simulink library "halout"  (R2021b)
settings: Solver=VariableStepAuto  StartTime=0.0  StopTime=10.0  RelTol=1e-3
undefined symbols (not defined in the file): C_TASK_5MS_S, FALSE, KHAL_CAN1TxReq_flg, KHAL_CAN2TxReq_flg, KHAL_CAN3FD3VCU1toNIDECTxReq_flg, KHAL_CAN3FD3VCU1TxReq_flg, KHAL_CAN3FD3VCU2E2E_flg, KHAL_CAN3FD3VCU2toNIDECE2E_flg, KHAL_CAN3FD3VCU2toNIDECTxReq_flg, KHAL_CAN3FD3VCU2TxReq_flg, KHAL_CAN3TxReq_flg, KHAL_CAN4FD4CE1000E2E_flg, KHAL_CAN4FD4CE1000TxReq_flg, KHAL_CAN4TxReq_flg, KHAL_CAN5TxReq_flg, KHAL_CAN7TxReq_flg, ONE_INT, TRUE, ZERO_INT
libraries: FVT_lib x258, simulink x115
(part 9 of 17)

== system halout/HAL_OUT/CAN5/FD5_CE100_0_0x118 ==
  BSCP_outputs : Inport  OutDataTypeStr=Bus: BSCP_outputs
  BOUTP_outputs : Inport  Port=2  OutDataTypeStr=Bus: BOUTP_outputs
  AllDoorSW : Subsystem
  AntitheftSta : Subsystem
  BCMDoorLockSta : Subsystem
  CCUACLampSts : Subsystem
  CCUCbnPreACWkSts : Subsystem
  CCUCbnPreEstimdTi : Subsystem
  CCUCbnPreSts : Subsystem
  FDTBOXDTCDataErr : Subsystem
  FDTBOXDTCDataSta : Subsystem
  FDTBOXVehDataErr : Subsystem
  FDTBOXVehDataSta : Subsystem
  Ground{,1..13} (14 alike) : Ground
  HoodSW : Subsystem
  LowSOCWarn : Subsystem
  PwrSta : Subsystem
  ReVehThdChkSta : Subsystem
  ShiftGearPosn : Subsystem
  TCountSta : Subsystem
  TailgateRemote : Subsystem
  TailgateSW : Subsystem
  VehMalfunLevel : Subsystem
  bus_creator : BusCreator  Inputs=20  OutDataTypeStr=Bus: DT_CAN5_SG_FD5_CE100_0  NonVirtualBus=on
  bus_selector : BusSelector  OutputSignals=VOUTP_CCUACLampSts_flg
  bus_selector1 : BusSelector  OutputSignals=VOUTP_LowSOCWarn_enum
  bus_selector2 : BusSelector  OutputSignals=VOUTP_PowerSta_enum
  bus_selector3 : BusSelector  OutputSignals=VOUTP_ReVehThdChkSta_enum
  bus_selector4 : BusSelector  OutputSignals=VOUTP_ShiftGearPosn_enum
  bus_selector5 : BusSelector  OutputSignals=VOUTP_TCountSta_enum
  FD5_CE100_0 : Outport
  wires:
  BSCP_outputs/1 -> [BSCP_outputs]
  BOUTP_outputs/1 -> [BOUTP_outputs]
  [CAN5_AllDoorSW] -> bus_creator/1  "CAN5_AllDoorSW"
  [CAN5_AntitheftSta] -> bus_creator/2  "CAN5_AntitheftSta"
  [CAN5_BCM_DoorLock_Sta] -> bus_creator/3  "CAN5_BCM_DoorLock_Sta"
  [CAN5_CCU_ACLampSts] -> bus_creator/4  "CAN5_CCU_ACLampSts"
  [CAN5_CCU_CbnPreACWkSts] -> bus_creator/5  "CAN5_CCU_CbnPreACWkSts"
  [CAN5_CCU_CbnPreEstimdTi] -> bus_creator/6  "CAN5_CCU_CbnPreEstimdTi"
  [CAN5_CCU_CbnPreSts] -> bus_creator/7  "CAN5_CCU_CbnPreSts"
  [CAN5_FD_TBOX_DTCData_Err] -> bus_creator/8  "CAN5_FD_TBOX_DTCData_Err"
  [CAN5_FD_TBOX_DTCData_Sta] -> bus_creator/9  "CAN5_FD_TBOX_DTCData_Sta"
  [CAN5_FD_TBOX_VehData_Err] -> bus_creator/10  "CAN5_FD_TBOX_VehData_Err"
  [CAN5_FD_TBOX_VehData_Sta] -> bus_creator/11  "CAN5_FD_TBOX_VehData_Sta"
  [CAN5_HoodSW] -> bus_creator/12  "CAN5_HoodSW"
  [CAN5_LowSOCWarn] -> bus_creator/13  "CAN5_LowSOCWarn"
  [CAN5_PwrSta] -> bus_creator/14  "CAN5_PwrSta"
  [CAN5_Re_VehThdChkSta] -> bus_creator/15  "CAN5_Re_VehThdChkSta"
  [CAN5_ShiftGearPosn] -> bus_creator/16  "CAN5_ShiftGearPosn"
  [CAN5_TCountSta] -> bus_creator/17  "CAN5_TCountSta"
  [CAN5_TailgateRemote] -> bus_creator/18  "CAN5_TailgateRemote"
  [CAN5_Tailgate_SW] -> bus_creator/19  "CAN5_Tailgate_SW"
  [CAN5_VehMalfunLevel] -> bus_creator/20  "CAN5_VehMalfunLevel"
  bus_creator/1 -> FD5_CE100_0/1
  AllDoorSW/1(CAN5_AllDoorSW) -> [CAN5_AllDoorSW]
  AntitheftSta/1(CAN5_AntitheftSta) -> [CAN5_AntitheftSta]
  BCMDoorLockSta/1(CAN5_BCM_DoorLock_Sta) -> [CAN5_BCM_DoorLock_Sta]
  CCUACLampSts/1(CAN5_CCU_ACLampSts) -> [CAN5_CCU_ACLampSts]
  CCUCbnPreACWkSts/1(CAN5_CCU_CbnPreACWkSts) -> [CAN5_CCU_CbnPreACWkSts]
  CCUCbnPreEstimdTi/1(CAN5_CCU_CbnPreEstimdTi) -> [CAN5_CCU_CbnPreEstimdTi]
  CCUCbnPreSts/1(CAN5_CCU_CbnPreSts) -> [CAN5_CCU_CbnPreSts]
  FDTBOXDTCDataErr/1(CAN5_FD_TBOX_DTCData_Err) -> [CAN5_FD_TBOX_DTCData_Err]
  FDTBOXDTCDataSta/1(CAN5_FD_TBOX_DTCData_Sta) -> [CAN5_FD_TBOX_DTCData_Sta]
  FDTBOXVehDataErr/1(CAN5_FD_TBOX_VehData_Err) -> [CAN5_FD_TBOX_VehData_Err]
  FDTBOXVehDataSta/1(CAN5_FD_TBOX_VehData_Sta) -> [CAN5_FD_TBOX_VehData_Sta]
  HoodSW/1(CAN5_HoodSW) -> [CAN5_HoodSW]
  LowSOCWarn/1(CAN5_LowSOCWarn) -> [CAN5_LowSOCWarn]
  PwrSta/1(CAN5_PwrSta) -> [CAN5_PwrSta]
  ReVehThdChkSta/1(CAN5_Re_VehThdChkSta) -> [CAN5_Re_VehThdChkSta]
  ShiftGearPosn/1(CAN5_ShiftGearPosn) -> [CAN5_ShiftGearPosn]
  TCountSta/1(CAN5_TCountSta) -> [CAN5_TCountSta]
  TailgateRemote/1(CAN5_TailgateRemote) -> [CAN5_TailgateRemote]
  TailgateSW/1(CAN5_Tailgate_SW) -> [CAN5_Tailgate_SW]
  VehMalfunLevel/1(CAN5_VehMalfunLevel) -> [CAN5_VehMalfunLevel]
  Ground/1 -> AllDoorSW/1(AllDoorSW)
  Ground1/1 -> AntitheftSta/1(AntitheftSta)
  Ground2/1 -> BCMDoorLockSta/1(BCMDoorLockSta)
  bus_selector/1 -> CCUACLampSts/1(CCUACLampSts)  "<VOUTP_CCUACLampSts_flg>"
  [BOUTP_outputs] -> bus_selector/1
  Ground3/1 -> CCUCbnPreACWkSts/1(CCUCbnPreACWkSts)
  Ground4/1 -> CCUCbnPreEstimdTi/1(CCUCbnPreEstimdTi)
  Ground5/1 -> CCUCbnPreSts/1(CCUCbnPreSts)
  Ground6/1 -> FDTBOXDTCDataErr/1(FDTBOXDTCDataErr)
  Ground7/1 -> FDTBOXDTCDataSta/1(FDTBOXDTCDataSta)
  Ground8/1 -> FDTBOXVehDataErr/1(FDTBOXVehDataErr)
  Ground9/1 -> FDTBOXVehDataSta/1(FDTBOXVehDataSta)
  Ground10/1 -> HoodSW/1(HoodSW)
  bus_selector1/1 -> LowSOCWarn/1(LowSOCWarn)  "<VOUTP_LowSOCWarn_enum>"
  [BOUTP_outputs] -> bus_selector1/1
  bus_selector2/1 -> PwrSta/1(PwrSta)  "<VOUTP_PowerSta_enum>"
  [BOUTP_outputs] -> bus_selector2/1
  bus_selector3/1 -> ReVehThdChkSta/1(ReVehThdChkSta)  "<VOUTP_ReVehThdChkSta_enum>"
  [BOUTP_outputs] -> bus_selector3/1
  bus_selector4/1 -> ShiftGearPosn/1(ShiftGearPosn)  "<VOUTP_ShiftGearPosn_enum>"
  [BOUTP_outputs] -> bus_selector4/1
  bus_selector5/1 -> TCountSta/1(TCountSta)  "<VOUTP_TCountSta_enum>"
  [BOUTP_outputs] -> bus_selector5/1
  Ground11/1 -> TailgateRemote/1(TailgateRemote)
  Ground12/1 -> TailgateSW/1(TailgateSW)
  Ground13/1 -> VehMalfunLevel/1(VehMalfunLevel)

== system halout/HAL_OUT/CAN5/FD5_Debug1_0x4D0 ==
  BSCP_outputs : Inport  OutDataTypeStr=Bus: BSCP_outputs
  BOUTP_outputs : Inport  Port=2  OutDataTypeStr=Bus: BOUTP_outputs
  ID1ALTU : Subsystem
  ID1LocALTU : Subsystem
  ID1messageALTU : Subsystem
  ID2ALTU : Subsystem
  ID2LocALTU : Subsystem
  ID2messageALTU : Subsystem
  ID3ALTU : Subsystem
  ID3LocALTU : Subsystem
  ID3messageALTU : Subsystem
  ID4ALTU : Subsystem
  ID4LocALTU : Subsystem
  ID4messageALTU : Subsystem
  IDinALTU : Subsystem
  LFSensorMode : Subsystem
  LRSensorMode : Subsystem
  RFFATALTU : Subsystem
  RFSensorMode : Subsystem
  RRSensorMode : Subsystem
  S1WheelDebugALTU : Subsystem
  S2WheelDebugALTU : Subsystem
  S3WheelDebugALTU : Subsystem
  S4WheelDebugALTU : Subsystem
  bus_creator : BusCreator  Inputs=22  OutDataTypeStr=Bus: DT_CAN5_SG_FD5_Debug1  NonVirtualBus=on
  bus_selector : BusSelector  OutputSignals=VOUTP_S1ID_raw32
  bus_selector1 : BusSelector  OutputSignals=VOUTP_S1L_enum
  bus_selector10 : BusSelector  OutputSignals=VOUTP_S4L_enum
  bus_selector11 : BusSelector  OutputSignals=VOUTP_ID4messageALTU_raw8
  bus_selector12 : BusSelector  OutputSignals=VOUTP_IDin_raw32
  bus_selector13 : BusSelector  OutputSignals=VOUTP_LFSensorMode_flg
  bus_selector14 : BusSelector  OutputSignals=VOUTP_LRSensorMode_flg
  bus_selector15 : BusSelector  OutputSignals=VOUTP_RFSensorMode_flg
  bus_selector16 : BusSelector  OutputSignals=VOUTP_FAT_flg
  bus_selector17 : BusSelector  OutputSignals=VOUTP_RRSensorMode_flg
  bus_selector18 : BusSelector  OutputSignals=VOUTP_S1WheelDebugALTU_pct
  bus_selector19 : BusSelector  OutputSignals=VOUTP_S2WheelDebugALTU_pct
  bus_selector2 : BusSelector  OutputSignals=VOUTP_ID1messageALTU_raw8
  bus_selector20 : BusSelector  OutputSignals=VOUTP_S3WheelDebugALTU_pct
  bus_selector21 : BusSelector  OutputSignals=VOUTP_S4WheelDebugALTU_pct
  bus_selector3 : BusSelector  OutputSignals=VOUTP_S2ID_raw32
  bus_selector4 : BusSelector  OutputSignals=VOUTP_S2L_enum
  bus_selector5 : BusSelector  OutputSignals=VOUTP_ID2messageALTU_raw8
  bus_selector6 : BusSelector  OutputSignals=VOUTP_S3ID_raw32
  bus_selector7 : BusSelector  OutputSignals=VOUTP_S3L_enum
  bus_selector8 : BusSelector  OutputSignals=VOUTP_ID3messageALTU_raw8
  bus_selector9 : BusSelector  OutputSignals=VOUTP_S4ID_raw32
  FD5_Debug1 : Outport
  wires:
  BSCP_outputs/1 -> [BSCP_outputs]
  BOUTP_outputs/1 -> [BOUTP_outputs]
  [CAN5_ID1_ALTU] -> bus_creator/1  "CAN5_ID1_ALTU"
  [CAN5_ID1_Loc_ALTU] -> bus_creator/2  "CAN5_ID1_Loc_ALTU"
  [CAN5_ID1_message_ALTU] -> bus_creator/3  "CAN5_ID1_message_ALTU"
  [CAN5_ID2_ALTU] -> bus_creator/4  "CAN5_ID2_ALTU"
  [CAN5_ID2_Loc_ALTU] -> bus_creator/5  "CAN5_ID2_Loc_ALTU"
  [CAN5_ID2_message_ALTU] -> bus_creator/6  "CAN5_ID2_message_ALTU"
  [CAN5_ID3_ALTU] -> bus_creator/7  "CAN5_ID3_ALTU"
  [CAN5_ID3_Loc_ALTU] -> bus_creator/8  "CAN5_ID3_Loc_ALTU"
  [CAN5_ID3_message_ALTU] -> bus_creator/9  "CAN5_ID3_message_ALTU"
  [CAN5_ID4_ALTU] -> bus_creator/10  "CAN5_ID4_ALTU"
  [CAN5_ID4_Loc_ALTU] -> bus_creator/11  "CAN5_ID4_Loc_ALTU"
  [CAN5_ID4_message_ALTU] -> bus_creator/12  "CAN5_ID4_message_ALTU"
  [CAN5_IDin_ALTU] -> bus_creator/13  "CAN5_IDin_ALTU"
  [CAN5_LFSensorMode] -> bus_creator/14  "CAN5_LFSensorMode"
  [CAN5_LRSensorMode] -> bus_creator/15  "CAN5_LRSensorMode"
  [CAN5_RFSensorMode] -> bus_creator/16  "CAN5_RFSensorMode"
  [CAN5_RF_FAT_ALTU] -> bus_creator/17  "CAN5_RF_FAT_ALTU"
  [CAN5_RRSensorMode] -> bus_creator/18  "CAN5_RRSensorMode"
  [CAN5_S1WheelDebug_ALTU] -> bus_creator/19  "CAN5_S1WheelDebug_ALTU"
  [CAN5_S2WheelDebug_ALTU] -> bus_creator/20  "CAN5_S2WheelDebug_ALTU"
  [CAN5_S3WheelDebug_ALTU] -> bus_creator/21  "CAN5_S3WheelDebug_ALTU"
  [CAN5_S4WheelDebug_ALTU] -> bus_creator/22  "CAN5_S4WheelDebug_ALTU"
  bus_creator/1 -> FD5_Debug1/1
  ID1ALTU/1(CAN5_ID1_ALTU) -> [CAN5_ID1_ALTU]
  ID1LocALTU/1(CAN5_ID1_Loc_ALTU) -> [CAN5_ID1_Loc_ALTU]
  ID1messageALTU/1(CAN5_ID1_message_ALTU) -> [CAN5_ID1_message_ALTU]
  ID2ALTU/1(CAN5_ID2_ALTU) -> [CAN5_ID2_ALTU]
  ID2LocALTU/1(CAN5_ID2_Loc_ALTU) -> [CAN5_ID2_Loc_ALTU]
  ID2messageALTU/1(CAN5_ID2_message_ALTU) -> [CAN5_ID2_message_ALTU]
  ID3ALTU/1(CAN5_ID3_ALTU) -> [CAN5_ID3_ALTU]
  ID3LocALTU/1(CAN5_ID3_Loc_ALTU) -> [CAN5_ID3_Loc_ALTU]
  ID3messageALTU/1(CAN5_ID3_message_ALTU) -> [CAN5_ID3_message_ALTU]
  ID4ALTU/1(CAN5_ID4_ALTU) -> [CAN5_ID4_ALTU]
  ID4LocALTU/1(CAN5_ID4_Loc_ALTU) -> [CAN5_ID4_Loc_ALTU]
  ID4messageALTU/1(CAN5_ID4_message_ALTU) -> [CAN5_ID4_message_ALTU]
  IDinALTU/1(CAN5_IDin_ALTU) -> [CAN5_IDin_ALTU]
  LFSensorMode/1(CAN5_LFSensorMode) -> [CAN5_LFSensorMode]
  LRSensorMode/1(CAN5_LRSensorMode) -> [CAN5_LRSensorMode]
  RFSensorMode/1(CAN5_RFSensorMode) -> [CAN5_RFSensorMode]
  RFFATALTU/1(CAN5_RF_FAT_ALTU) -> [CAN5_RF_FAT_ALTU]
  RRSensorMode/1(CAN5_RRSensorMode) -> [CAN5_RRSensorMode]
  S1WheelDebugALTU/1(CAN5_S1WheelDebug_ALTU) -> [CAN5_S1WheelDebug_ALTU]
  S2WheelDebugALTU/1(CAN5_S2WheelDebug_ALTU) -> [CAN5_S2WheelDebug_ALTU]
  S3WheelDebugALTU/1(CAN5_S3WheelDebug_ALTU) -> [CAN5_S3WheelDebug_ALTU]
  S4WheelDebugALTU/1(CAN5_S4WheelDebug_ALTU) -> [CAN5_S4WheelDebug_ALTU]
  bus_selector/1 -> ID1ALTU/1(ID1ALTU)  "<VOUTP_S1ID_raw32>"
  [BOUTP_outputs] -> bus_selector/1
  bus_selector1/1 -> ID1LocALTU/1(ID1LocALTU)  "<VOUTP_S1L_enum>"
  [BOUTP_outputs] -> bus_selector1/1
  bus_selector2/1 -> ID1messageALTU/1(ID1messageALTU)  "<VOUTP_ID1messageALTU_raw8>"
  [BOUTP_outputs] -> bus_selector2/1
  bus_selector3/1 -> ID2ALTU/1(ID2ALTU)  "<VOUTP_S2ID_raw32>"
  [BOUTP_outputs] -> bus_selector3/1
  bus_selector4/1 -> ID2LocALTU/1(ID2LocALTU)  "<VOUTP_S2L_enum>"
  [BOUTP_outputs] -> bus_selector4/1
  bus_selector5/1 -> ID2messageALTU/1(ID2messageALTU)  "<VOUTP_ID2messageALTU_raw8>"
  [BOUTP_outputs] -> bus_selector5/1
  bus_selector6/1 -> ID3ALTU/1(ID3ALTU)  "<VOUTP_S3ID_raw32>"
  [BOUTP_outputs] -> bus_selector6/1
  bus_selector7/1 -> ID3LocALTU/1(ID3LocALTU)  "<VOUTP_S3L_enum>"
  [BOUTP_outputs] -> bus_selector7/1
  bus_selector8/1 -> ID3messageALTU/1(ID3messageALTU)  "<VOUTP_ID3messageALTU_raw8>"
  [BOUTP_outputs] -> bus_selector8/1
  bus_selector9/1 -> ID4ALTU/1(ID4ALTU)  "<VOUTP_S4ID_raw32>"
  [BOUTP_outputs] -> bus_selector9/1
  bus_selector10/1 -> ID4LocALTU/1(ID4LocALTU)  "<VOUTP_S4L_enum>"
  [BOUTP_outputs] -> bus_selector10/1
  bus_selector11/1 -> ID4messageALTU/1(ID4messageALTU)  "<VOUTP_ID4messageALTU_raw8>"
  [BOUTP_outputs] -> bus_selector11/1
  bus_selector12/1 -> IDinALTU/1(IDinALTU)  "<VOUTP_IDin_raw32>"
  [BOUTP_outputs] -> bus_selector12/1
  bus_selector13/1 -> LFSensorMode/1(LFSensorMode)  "<VOUTP_LFSensorMode_flg>"
  [BOUTP_outputs] -> bus_selector13/1
  bus_selector14/1 -> LRSensorMode/1(LRSensorMode)  "<VOUTP_LRSensorMode_flg>"
  [BOUTP_outputs] -> bus_selector14/1
  bus_selector15/1 -> RFSensorMode/1(RFSensorMode)  "<VOUTP_RFSensorMode_flg>"
  [BOUTP_outputs] -> bus_selector15/1
  bus_selector16/1 -> RFFATALTU/1(RFFATALTU)  "<VOUTP_FAT_flg>"
  [BOUTP_outputs] -> bus_selector16/1
  bus_selector17/1 -> RRSensorMode/1(RRSensorMode)  "<VOUTP_RRSensorMode_flg>"
  [BOUTP_outputs] -> bus_selector17/1
  bus_selector18/1 -> S1WheelDebugALTU/1(S1WheelDebugALTU)  "<VOUTP_S1WheelDebugALTU_pct>"
  [BOUTP_outputs] -> bus_selector18/1
  bus_selector19/1 -> S2WheelDebugALTU/1(S2WheelDebugALTU)  "<VOUTP_S2WheelDebugALTU_pct>"
  [BOUTP_outputs] -> bus_selector19/1
  bus_selector20/1 -> S3WheelDebugALTU/1(S3WheelDebugALTU)  "<VOUTP_S3WheelDebugALTU_pct>"
  [BOUTP_outputs] -> bus_selector20/1
  bus_selector21/1 -> S4WheelDebugALTU/1(S4WheelDebugALTU)  "<VOUTP_S4WheelDebugALTU_pct>"
  [BOUTP_outputs] -> bus_selector21/1

== system halout/HAL_OUT/CAN5/GW5_CE100_0_0x1C5 ==
  BSCP_outputs : Inport  OutDataTypeStr=Bus: BSCP_outputs
  BOUTP_outputs : Inport  Port=2  OutDataTypeStr=Bus: BOUTP_outputs
  BrkSwSta : Subsystem
  CrashOutputSts : Subsystem
  Ground{,1..10} (11 alike) : Ground
  PTGActiveSta : Subsystem
  PTGExist : Subsystem
  PTGSysSta : Subsystem
  VehSpeed : Subsystem
  ZLAPMWinLFOpenedSta : Subsystem
  ZLAPMWinLROpenedSta : Subsystem
  ZRAPMWinRFOpenedSta : Subsystem
  ZRAPMWinRROpenedSta : Subsystem
  ZRPTGActiveSta : Subsystem
  ZRPTGExistSta : Subsystem
  ZRPTGSysSta : Subsystem
  bus_creator : BusCreator  Inputs=13  OutDataTypeStr=Bus: DT_CAN5_SG_GW5_CE100_0  NonVirtualBus=on
  bus_selector : BusSelector  OutputSignals=VOUTP_SCPBrkSwSta_flg
  bus_selector1 : BusSelector  OutputSignals=VOUTP_Vehspeed_kph
  GW5_CE100_0 : Outport
  wires:
  BSCP_outputs/1 -> [BSCP_outputs]
  BOUTP_outputs/1 -> [BOUTP_outputs]
  [CAN5_BrkSw_Sta] -> bus_creator/1  "CAN5_BrkSw_Sta"
  [CAN5_CrashOutputSts] -> bus_creator/2  "CAN5_CrashOutputSts"
  [CAN5_PTG_Active_Sta] -> bus_creator/3  "CAN5_PTG_Active_Sta"
  [CAN5_PTG_Exist] -> bus_creator/4  "CAN5_PTG_Exist"
  [CAN5_PTG_Sys_Sta] -> bus_creator/5  "CAN5_PTG_Sys_Sta"
  [CAN5_VehSpeed] -> bus_creator/6  "CAN5_VehSpeed"
  [CAN5_ZL_APM_WinLFOpened_Sta] -> bus_creator/7  "CAN5_ZL_APM_WinLFOpened_Sta"
  [CAN5_ZL_APM_WinLROpened_Sta] -> bus_creator/8  "CAN5_ZL_APM_WinLROpened_Sta"
  [CAN5_ZR_APM_WinRFOpened_Sta] -> bus_creator/9  "CAN5_ZR_APM_WinRFOpened_Sta"
  [CAN5_ZR_APM_WinRROpened_Sta] -> bus_creator/10  "CAN5_ZR_APM_WinRROpened_Sta"
  [CAN5_ZR_PTG_Active_Sta] -> bus_creator/11  "CAN5_ZR_PTG_Active_Sta"
  [CAN5_ZR_PTG_Exist_Sta] -> bus_creator/12  "CAN5_ZR_PTG_Exist_Sta"
  [CAN5_ZR_PTG_Sys_Sta] -> bus_creator/13  "CAN5_ZR_PTG_Sys_Sta"
  bus_creator/1 -> GW5_CE100_0/1
  BrkSwSta/1(CAN5_BrkSw_Sta) -> [CAN5_BrkSw_Sta]
  CrashOutputSts/1(CAN5_CrashOutputSts) -> [CAN5_CrashOutputSts]
  PTGActiveSta/1(CAN5_PTG_Active_Sta) -> [CAN5_PTG_Active_Sta]
  PTGExist/1(CAN5_PTG_Exist) -> [CAN5_PTG_Exist]
  PTGSysSta/1(CAN5_PTG_Sys_Sta) -> [CAN5_PTG_Sys_Sta]
  VehSpeed/1(CAN5_VehSpeed) -> [CAN5_VehSpeed]
  ZLAPMWinLFOpenedSta/1(CAN5_ZL_APM_WinLFOpened_Sta) -> [CAN5_ZL_APM_WinLFOpened_Sta]
  ZLAPMWinLROpenedSta/1(CAN5_ZL_APM_WinLROpened_Sta) -> [CAN5_ZL_APM_WinLROpened_Sta]
  ZRAPMWinRFOpenedSta/1(CAN5_ZR_APM_WinRFOpened_Sta) -> [CAN5_ZR_APM_WinRFOpened_Sta]
  ZRAPMWinRROpenedSta/1(CAN5_ZR_APM_WinRROpened_Sta) -> [CAN5_ZR_APM_WinRROpened_Sta]
  ZRPTGActiveSta/1(CAN5_ZR_PTG_Active_Sta) -> [CAN5_ZR_PTG_Active_Sta]
  ZRPTGExistSta/1(CAN5_ZR_PTG_Exist_Sta) -> [CAN5_ZR_PTG_Exist_Sta]
  ZRPTGSysSta/1(CAN5_ZR_PTG_Sys_Sta) -> [CAN5_ZR_PTG_Sys_Sta]
  bus_selector/1 -> BrkSwSta/1(BrkSwSta)  "<VOUTP_SCPBrkSwSta_flg>"
  [BOUTP_outputs] -> bus_selector/1
  Ground/1 -> CrashOutputSts/1(CrashOutputSts)
  Ground1/1 -> PTGActiveSta/1(PTGActiveSta)
  Ground2/1 -> PTGExist/1(PTGExist)
  Ground3/1 -> PTGSysSta/1(PTGSysSta)
  bus_selector1/1 -> VehSpeed/1(VehSpeed)  "<VOUTP_Vehspeed_kph>"
  [BOUTP_outputs] -> bus_selector1/1
  Ground4/1 -> ZLAPMWinLFOpenedSta/1(ZLAPMWinLFOpenedSta)
  Ground5/1 -> ZLAPMWinLROpenedSta/1(ZLAPMWinLROpenedSta)
  Ground6/1 -> ZRAPMWinRFOpenedSta/1(ZRAPMWinRFOpenedSta)
  Ground7/1 -> ZRAPMWinRROpenedSta/1(ZRAPMWinRROpenedSta)
  Ground8/1 -> ZRPTGActiveSta/1(ZRPTGActiveSta)
  Ground9/1 -> ZRPTGExistSta/1(ZRPTGExistSta)
  Ground10/1 -> ZRPTGSysSta/1(ZRPTGSysSta)

== system halout/HAL_OUT/CAN7/FD7_CE100_0_0x18FA05B9 ==
  BSCP_outputs : Inport  OutDataTypeStr=Bus: BSCP_outputs
  BOUTP_outputs : Inport  Port=2  OutDataTypeStr=Bus: BOUTP_outputs
  FDCBCMFDDoorOpenSta : Subsystem
  LTurnLP : Subsystem
  RTurnLP : Subsystem
  bus_creator : BusCreator  Inputs=3  OutDataTypeStr=Bus: DT_CAN7_SG_FD7_CE100_0  NonVirtualBus=on
  bus_selector : BusSelector  OutputSignals=VOUTP_FDDoorOpen_enum
  bus_selector1 : BusSelector  OutputSignals=VOUTP_LTurnLP_flg
  bus_selector2 : BusSelector  OutputSignals=VOUTP_RTurnLP_flg
  FD7_CE100_0 : Outport
  wires:
  BSCP_outputs/1 -> [BSCP_outputs]
  BOUTP_outputs/1 -> [BOUTP_outputs]
  [CAN7_FDC_BCM_FDDoorOpen_Sta] -> bus_creator/1  "CAN7_FDC_BCM_FDDoorOpen_Sta"
  [CAN7_LTurnLP] -> bus_creator/2  "CAN7_LTurnLP"
  [CAN7_RTurnLP] -> bus_creator/3  "CAN7_RTurnLP"
  bus_creator/1 -> FD7_CE100_0/1
  FDCBCMFDDoorOpenSta/1(CAN7_FDC_BCM_FDDoorOpen_Sta) -> [CAN7_FDC_BCM_FDDoorOpen_Sta]
  LTurnLP/1(CAN7_LTurnLP) -> [CAN7_LTurnLP]
  RTurnLP/1(CAN7_RTurnLP) -> [CAN7_RTurnLP]
  bus_selector/1 -> FDCBCMFDDoorOpenSta/1(FDCBCMFDDoorOpenSta)  "<VOUTP_FDDoorOpen_enum>"
  [BOUTP_outputs] -> bus_selector/1
  bus_selector1/1 -> LTurnLP/1(LTurnLP)  "<VOUTP_LTurnLP_flg>"
  [BOUTP_outputs] -> bus_selector1/1
  bus_selector2/1 -> RTurnLP/1(RTurnLP)  "<VOUTP_RTurnLP_flg>"
  [BOUTP_outputs] -> bus_selector2/1

== system halout/HAL_OUT/CAN7/FD7_CE100_1_0xCFFE632 ==
  BSCP_outputs : Inport  OutDataTypeStr=Bus: BSCP_outputs
  BOUTP_outputs : Inport  Port=2  OutDataTypeStr=Bus: BOUTP_outputs
  FDCBCMFRClosedoorCmd : Subsystem
  FDCBCMFRHaltBrakeSta : Subsystem
  FDCBCMFROpenClosePBCmd : Subsystem
  FDCBCMFROpendoorCmd : Subsystem
  FDCBCMPosLampCmd : Subsystem
  FDCFRDisIntEmCmd : Subsystem
  Ground : Ground
  Ground1 : Ground
  Ground2 : Ground
  bus_creator : BusCreator  Inputs=6  OutDataTypeStr=Bus: DT_CAN7_SG_FD7_CE100_1  NonVirtualBus=on
  bus_selector : BusSelector  OutputSignals=VOUTP_FRHaltBrakeSta_enum
  bus_selector1 : BusSelector  OutputSignals=VOUTP_FROpenClosePBCmd_enum
  bus_selector2 : BusSelector  OutputSignals=VOUTP_PosLamp_flg
  FD7_CE100_1 : Outport
  wires:
  BSCP_outputs/1 -> [BSCP_outputs]
  BOUTP_outputs/1 -> [BOUTP_outputs]
  [CAN7_FDC_BCM_FRClosedoor_Cmd] -> bus_creator/1  "CAN7_FDC_BCM_FRClosedoor_Cmd"
  [CAN7_FDC_BCM_FRHaltBrake_Sta] -> bus_creator/2  "CAN7_FDC_BCM_FRHaltBrake_Sta"
  [CAN7_FDC_BCM_FROpenClosePB_Cmd] -> bus_creator/3  "CAN7_FDC_BCM_FROpenClosePB_Cmd"
  [CAN7_FDC_BCM_FROpendoor_Cmd] -> bus_creator/4  "CAN7_FDC_BCM_FROpendoor_Cmd"
  [CAN7_FDC_BCM_PosLamp_Cmd] -> bus_creator/5  "CAN7_FDC_BCM_PosLamp_Cmd"
  [CAN7_FDC_FRDisIntEm_Cmd] -> bus_creator/6  "CAN7_FDC_FRDisIntEm_Cmd"
  bus_creator/1 -> FD7_CE100_1/1
  FDCBCMFRClosedoorCmd/1(CAN7_FDC_BCM_FRClosedoor_Cmd) -> [CAN7_FDC_BCM_FRClosedoor_Cmd]
  FDCBCMFRHaltBrakeSta/1(CAN7_FDC_BCM_FRHaltBrake_Sta) -> [CAN7_FDC_BCM_FRHaltBrake_Sta]
  FDCBCMFROpenClosePBCmd/1(CAN7_FDC_BCM_FROpenClosePB_Cmd) -> [CAN7_FDC_BCM_FROpenClosePB_Cmd]
  FDCBCMFROpendoorCmd/1(CAN7_FDC_BCM_FROpendoor_Cmd) -> [CAN7_FDC_BCM_FROpendoor_Cmd]
  FDCBCMPosLampCmd/1(CAN7_FDC_BCM_PosLamp_Cmd) -> [CAN7_FDC_BCM_PosLamp_Cmd]
  FDCFRDisIntEmCmd/1(CAN7_FDC_FRDisIntEm_Cmd) -> [CAN7_FDC_FRDisIntEm_Cmd]
  Ground/1 -> FDCBCMFRClosedoorCmd/1(FDCBCMFRClosedoorCmd)
  bus_selector/1 -> FDCBCMFRHaltBrakeSta/1(FDCBCMFRHaltBrakeSta)  "<VOUTP_FRHaltBrakeSta_enum>"
  [BOUTP_outputs] -> bus_selector/1
  bus_selector1/1 -> FDCBCMFROpenClosePBCmd/1(FDCBCMFROpenClosePBCmd)  "<VOUTP_FROpenClosePBCmd_enum>"
  [BOUTP_outputs] -> bus_selector1/1
  Ground1/1 -> FDCBCMFROpendoorCmd/1(FDCBCMFROpendoorCmd)
  bus_selector2/1 -> FDCBCMPosLampCmd/1(FDCBCMPosLampCmd)  "<VOUTP_PosLamp_flg>"
  [BOUTP_outputs] -> bus_selector2/1
  Ground2/1 -> FDCFRDisIntEmCmd/1(FDCFRDisIntEmCmd)

== system halout/HAL_OUT/CAN1/CCVS_0x18FEF100/BrakeSW ==
  BrakeSW : Inport
  Data Type Conversion : DataTypeConversion  OutDataTypeStr=uint8  RndMeth=Round
  CAN1_BrakeSW : Outport
  wires:
  Data Type Conversion/1 -> CAN1_BrakeSW/1
  BrakeSW/1 -> Data Type Conversion/1

== system halout/HAL_OUT/CAN1/CCVS_0x18FEF100/ParkBrakeSW ==
  ParkBrakeSW : Inport
  Data Type Conversion : DataTypeConversion  OutDataTypeStr=uint8  RndMeth=Round
  CAN1_ParkBrakeSW : Outport
  wires:
  Data Type Conversion/1 -> CAN1_ParkBrakeSW/1
  ParkBrakeSW/1 -> Data Type Conversion/1

== system halout/HAL_OUT/CAN1/CCVS_0x18FEF100/VCUVehSpd ==
  VCUVehSpd : Inport
  Data Type Conversion : DataTypeConversion  OutDataTypeStr=uint16  RndMeth=Round
  convert_out : FVT_lib/hal/convert_out  gain=0.0039062  offset=0
  CAN1_VCUVehSpd : Outport
  wires:
  Data Type Conversion/1 -> CAN1_VCUVehSpd/1
  convert_out/1 -> Data Type Conversion/1
  VCUVehSpd/1 -> convert_out/1

== system halout/HAL_OUT/CAN1/CFGEM1_BAM_0x18ECFFEF/CFGEM1BAMPGN ==
  CFGEM1BAMPGN : Inport
  Data Type Conversion : DataTypeConversion  OutDataTypeStr=uint32  RndMeth=Round
  CAN1_CFGEM1BAMPGN : Outport
  wires:
  Data Type Conversion/1 -> CAN1_CFGEM1BAMPGN/1
  CFGEM1BAMPGN/1 -> Data Type Conversion/1

== system halout/HAL_OUT/CAN1/CFGEM1_BAM_0x18ECFFEF/CFGEM1BAMRsv ==
  CFGEM1BAMRsv : Inport
  Data Type Conversion : DataTypeConversion  OutDataTypeStr=uint8  RndMeth=Round
  CAN1_CFGEM1BAMRsv : Outport
  wires:
  Data Type Conversion/1 -> CAN1_CFGEM1BAMRsv/1
  CFGEM1BAMRsv/1 -> Data Type Conversion/1

== system halout/HAL_OUT/CAN1/CFGEM1_BAM_0x18ECFFEF/CFGEM1BAMTNum ==
  CFGEM1BAMTNum : Inport
  Data Type Conversion : DataTypeConversion  OutDataTypeStr=uint8  RndMeth=Round
  CAN1_CFGEM1BAMTNum : Outport
  wires:
  Data Type Conversion/1 -> CAN1_CFGEM1BAMTNum/1
  CFGEM1BAMTNum/1 -> Data Type Conversion/1

== system halout/HAL_OUT/CAN1/CFGEM1_BAM_0x18ECFFEF/CFGEM1BAMTSize ==
  CFGEM1BAMTSize : Inport
  Data Type Conversion : DataTypeConversion  OutDataTypeStr=uint16  RndMeth=Round
  CAN1_CFGEM1BAMTSize : Outport
  wires:
  Data Type Conversion/1 -> CAN1_CFGEM1BAMTSize/1
  CFGEM1BAMTSize/1 -> Data Type Conversion/1

== system halout/HAL_OUT/CAN1/CFGEM1_BAM_0x18ECFFEF/CFGEM1Ctrl ==
  CFGEM1Ctrl : Inport
  Data Type Conversion : DataTypeConversion  OutDataTypeStr=uint8  RndMeth=Round
  CAN1_CFGEM1Ctrl : Outport
  wires:
  Data Type Conversion/1 -> CAN1_CFGEM1Ctrl/1
  CFGEM1Ctrl/1 -> Data Type Conversion/1

== system halout/HAL_OUT/CAN1/CFGEM1_DT_0x18EBFFEF/CFGEM1DT0 ==
  CFGEM1DT0 : Inport
  Data Type Conversion : DataTypeConversion  OutDataTypeStr=uint8  RndMeth=Round
  CAN1_CFGEM1DT0 : Outport
  wires:
  Data Type Conversion/1 -> CAN1_CFGEM1DT0/1
  CFGEM1DT0/1 -> Data Type Conversion/1

== system halout/HAL_OUT/CAN1/CFGEM1_DT_0x18EBFFEF/CFGEM1DT1 ==
  CFGEM1DT1 : Inport
  Data Type Conversion : DataTypeConversion  OutDataTypeStr=uint8  RndMeth=Round
  CAN1_CFGEM1DT1 : Outport
  wires:
  Data Type Conversion/1 -> CAN1_CFGEM1DT1/1
  CFGEM1DT1/1 -> Data Type Conversion/1

== system halout/HAL_OUT/CAN1/CFGEM1_DT_0x18EBFFEF/CFGEM1DT2 ==
  CFGEM1DT2 : Inport
  Data Type Conversion : DataTypeConversion  OutDataTypeStr=uint8  RndMeth=Round
  CAN1_CFGEM1DT2 : Outport
  wires:
  Data Type Conversion/1 -> CAN1_CFGEM1DT2/1
  CFGEM1DT2/1 -> Data Type Conversion/1

== system halout/HAL_OUT/CAN1/CFGEM1_DT_0x18EBFFEF/CFGEM1DT3 ==
  CFGEM1DT3 : Inport
  Data Type Conversion : DataTypeConversion  OutDataTypeStr=uint8  RndMeth=Round
  CAN1_CFGEM1DT3 : Outport
  wires:
  Data Type Conversion/1 -> CAN1_CFGEM1DT3/1
  CFGEM1DT3/1 -> Data Type Conversion/1

== system halout/HAL_OUT/CAN1/CFGEM1_DT_0x18EBFFEF/CFGEM1DT4 ==
  CFGEM1DT4 : Inport
  Data Type Conversion : DataTypeConversion  OutDataTypeStr=uint8  RndMeth=Round
  CAN1_CFGEM1DT4 : Outport
  wires:
  Data Type Conversion/1 -> CAN1_CFGEM1DT4/1
  CFGEM1DT4/1 -> Data Type Conversion/1

== system halout/HAL_OUT/CAN1/CFGEM1_DT_0x18EBFFEF/CFGEM1DT5 ==
  CFGEM1DT5 : Inport
  Data Type Conversion : DataTypeConversion  OutDataTypeStr=uint8  RndMeth=Round
  CAN1_CFGEM1DT5 : Outport
  wires:
  Data Type Conversion/1 -> CAN1_CFGEM1DT5/1
  CFGEM1DT5/1 -> Data Type Conversion/1

== system halout/HAL_OUT/CAN1/CFGEM1_DT_0x18EBFFEF/CFGEM1DT6 ==
  CFGEM1DT6 : Inport
  Data Type Conversion : DataTypeConversion  OutDataTypeStr=uint8  RndMeth=Round
  CAN1_CFGEM1DT6 : Outport
  wires:
  Data Type Conversion/1 -> CAN1_CFGEM1DT6/1
  CFGEM1DT6/1 -> Data Type Conversion/1

== system halout/HAL_OUT/CAN1/CFGEM1_DT_0x18EBFFEF/CFGEM1DT7 ==
  CFGEM1DT7 : Inport
  Data Type Conversion : DataTypeConversion  OutDataTypeStr=uint8  RndMeth=Round
  CAN1_CFGEM1DT7 : Outport
  wires:
  Data Type Conversion/1 -> CAN1_CFGEM1DT7/1
  CFGEM1DT7/1 -> Data Type Conversion/1

== system halout/HAL_OUT/CAN1/EEC2_0xCF00300/AccPedal1LowSW ==
  AccPedal1LowSW : Inport
  Data Type Conversion : DataTypeConversion  OutDataTypeStr=uint8  RndMeth=Round
  CAN1_AccPedal1LowSW : Outport
  wires:
  Data Type Conversion/1 -> CAN1_AccPedal1LowSW/1
  AccPedal1LowSW/1 -> Data Type Conversion/1

== system halout/HAL_OUT/CAN1/EEC2_0xCF00300/AccPedalPos1 ==
  AccPedalPos1 : Inport
  Data Type Conversion : DataTypeConversion  OutDataTypeStr=uint8  RndMeth=Round
  convert_out : FVT_lib/hal/convert_out  gain=0.4  offset=0
  CAN1_AccPedalPos1 : Outport
  wires:
  Data Type Conversion/1 -> CAN1_AccPedalPos1/1
  convert_out/1 -> Data Type Conversion/1
  AccPedalPos1/1 -> convert_out/1

== system halout/HAL_OUT/CAN1/EEC2_0xCF00300/EEC2MSGCS ==
  EEC2MSGCS : Inport
  Data Type Conversion : DataTypeConversion  OutDataTypeStr=uint8  RndMeth=Round
  CAN1_EEC2MSGCS : Outport
  wires:
  Data Type Conversion/1 -> CAN1_EEC2MSGCS/1
  EEC2MSGCS/1 -> Data Type Conversion/1

== system halout/HAL_OUT/CAN1/EEC2_0xCF00300/EEC2MSGCnt ==
  EEC2MSGCnt : Inport
  Data Type Conversion : DataTypeConversion  OutDataTypeStr=uint8  RndMeth=Round
  CAN1_EEC2MSGCnt : Outport
  wires:
  Data Type Conversion/1 -> CAN1_EEC2MSGCnt/1
  EEC2MSGCnt/1 -> Data Type Conversion/1

== system halout/HAL_OUT/CAN1/EEC3_0x18FEDFEF/EMParasLoss ==
  EMParasLoss : Inport
  Data Type Conversion : DataTypeConversion  OutDataTypeStr=uint8  RndMeth=Round
  convert_out : FVT_lib/hal/convert_out  gain=1  offset=-125
  CAN1_EMParasLoss : Outport
  wires:
  Data Type Conversion/1 -> CAN1_EMParasLoss/1
  convert_out/1 -> Data Type Conversion/1
  EMParasLoss/1 -> convert_out/1

== system halout/HAL_OUT/CAN1/EEC3_0x18FEDFEF/NFricPercTorq ==
  NFricPercTorq : Inport
  Data Type Conversion : DataTypeConversion  OutDataTypeStr=uint8  RndMeth=Round
  convert_out : FVT_lib/hal/convert_out  gain=1  offset=-125
  CAN1_NFricPercTorq : Outport
  wires:
  Data Type Conversion/1 -> CAN1_NFricPercTorq/1
  convert_out/1 -> Data Type Conversion/1
  NFricPercTorq/1 -> convert_out/1

== system halout/HAL_OUT/CAN1/EMRC1_0x18FF20EF/ActEMOutSftSpd ==
  ActEMOutSftSpd : Inport
  Data Type Conversion : DataTypeConversion  OutDataTypeStr=uint16  RndMeth=Round
  convert_out : FVT_lib/hal/convert_out  gain=0.25  offset=0
  CAN1_ActEMOutSftSpd : Outport
  wires:
  Data Type Conversion/1 -> CAN1_ActEMOutSftSpd/1
  convert_out/1 -> Data Type Conversion/1
  ActEMOutSftSpd/1 -> convert_out/1

== system halout/HAL_OUT/CAN1/EMRC1_0x18FF20EF/ActEMpTrq ==
  ActEMpTrq : Inport
  Data Type Conversion : DataTypeConversion  OutDataTypeStr=uint8  RndMeth=Round
  convert_out : FVT_lib/hal/convert_out  gain=1  offset=-125
  CAN1_ActEMpTrq : Outport
  wires:
  Data Type Conversion/1 -> CAN1_ActEMpTrq/1
  convert_out/1 -> Data Type Conversion/1
  ActEMpTrq/1 -> convert_out/1

== system halout/HAL_OUT/CAN1/EMRC1_0x18FF20EF/ActEMpTrqHrls ==
  ActEMpTrqHrls : Inport
  Data Type Conversion : DataTypeConversion  OutDataTypeStr=uint8  RndMeth=Round
  convert_out : FVT_lib/hal/convert_out  gain=0.125  offset=0
  CAN1_ActEMpTrqHrls : Outport
  wires:
  Data Type Conversion/1 -> CAN1_ActEMpTrqHrls/1
  convert_out/1 -> Data Type Conversion/1
  ActEMpTrqHrls/1 -> convert_out/1

== system halout/HAL_OUT/CAN1/EMRC1_0x18FF20EF/ActMaxAvaEMRecpTrq ==
  ActMaxAvaEMRecpTrq : Inport
  Data Type Conversion : DataTypeConversion  OutDataTypeStr=uint8  RndMeth=Round
  convert_out : FVT_lib/hal/convert_out  gain=1  offset=-125
  CAN1_ActMaxAvaEMRecpTrq : Outport
  wires:
  Data Type Conversion/1 -> CAN1_ActMaxAvaEMRecpTrq/1
  convert_out/1 -> Data Type Conversion/1
  ActMaxAvaEMRecpTrq/1 -> convert_out/1

== system halout/HAL_OUT/CAN1/EMRC1_0x18FF20EF/DrvDemEMRtapTrq ==
  DrvDemEMRtapTrq : Inport
  Data Type Conversion : DataTypeConversion  OutDataTypeStr=uint8  RndMeth=Round
  convert_out : FVT_lib/hal/convert_out  gain=1  offset=-125
  CAN1_DrvDemEMRtapTrq : Outport
  wires:
  Data Type Conversion/1 -> CAN1_DrvDemEMRtapTrq/1
  convert_out/1 -> Data Type Conversion/1
  DrvDemEMRtapTrq/1 -> convert_out/1

== system halout/HAL_OUT/CAN1/EMRC1_0x18FF20EF/EMTrqModeDrvBrk ==
  EMTrqModeDrvBrk : Inport
  Data Type Conversion : DataTypeConversion  OutDataTypeStr=uint8  RndMeth=Round
  CAN1_EMTrqModeDrvBrk : Outport
  wires:
  Data Type Conversion/1 -> CAN1_EMTrqModeDrvBrk/1
  EMTrqModeDrvBrk/1 -> Data Type Conversion/1

== system halout/HAL_OUT/CAN1/EMRC1_0x18FF20EF/RetSelNonEng ==
  RetSelNonEng : Inport
  Data Type Conversion : DataTypeConversion  OutDataTypeStr=uint8  RndMeth=Round
  convert_out : FVT_lib/hal/convert_out  gain=0.4  offset=0
  CAN1_RetSelNonEng : Outport
  wires:
  Data Type Conversion/1 -> CAN1_RetSelNonEng/1
  convert_out/1 -> Data Type Conversion/1
  RetSelNonEng/1 -> convert_out/1

== system halout/HAL_OUT/CAN1/EMRC1_0x18FF20EF/SACtrlDev ==
  SACtrlDev : Inport
  Data Type Conversion : DataTypeConversion  OutDataTypeStr=uint8  RndMeth=Round
  CAN1_SACtrlDev : Outport
  wires:
  Data Type Conversion/1 -> CAN1_SACtrlDev/1
  SACtrlDev/1 -> Data Type Conversion/1

== system halout/HAL_OUT/CAN1/ETC1_0x18F00203/DLEngaged ==
  DLEngaged : Inport
  Data Type Conversion : DataTypeConversion  OutDataTypeStr=uint8  RndMeth=Round
  CAN1_DLEngaged : Outport
  wires:
  Data Type Conversion/1 -> CAN1_DLEngaged/1
  DLEngaged/1 -> Data Type Conversion/1

== system halout/HAL_OUT/CAN1/ETC1_0x18F00203/ShiftPgs ==
  ShiftPgs : Inport
  Data Type Conversion : DataTypeConversion  OutDataTypeStr=uint8  RndMeth=Round
  CAN1_ShiftPgs : Outport
  wires:
  Data Type Conversion/1 -> CAN1_ShiftPgs/1
  ShiftPgs/1 -> Data Type Conversion/1

== system halout/HAL_OUT/CAN1/ETC2_0x18F00503/ActDriveDirect ==
  ActDriveDirect : Inport
  Data Type Conversion : DataTypeConversion  OutDataTypeStr=uint8  RndMeth=Round
  convert_out : FVT_lib/hal/convert_out  gain=1  offset=-125
  CAN1_ActDriveDirect : Outport
  wires:
  Data Type Conversion/1 -> CAN1_ActDriveDirect/1
  convert_out/1 -> Data Type Conversion/1
  ActDriveDirect/1 -> convert_out/1

== system halout/HAL_OUT/CAN1/FD1_C100_1_0x18FF602B/FDCCHAEBSHBSwSta ==
  FDCCHAEBSHBSwSta : Inport
  Data Type Conversion : DataTypeConversion  OutDataTypeStr=uint8  RndMeth=Round
  CAN1_FDC_CHA_EBSHBSw_Sta : Outport
  wires:
  Data Type Conversion/1 -> CAN1_FDC_CHA_EBSHBSw_Sta/1
  FDCCHAEBSHBSwSta/1 -> Data Type Conversion/1

== system halout/HAL_OUT/CAN1/FD1_C100_1_0x18FF602B/FDCCHAEBSHHSwSta ==
  FDCCHAEBSHHSwSta : Inport
  Data Type Conversion : DataTypeConversion  OutDataTypeStr=uint8  RndMeth=Round
  CAN1_FDC_CHA_EBSHHSw_Sta : Outport
  wires:
  Data Type Conversion/1 -> CAN1_FDC_CHA_EBSHHSw_Sta/1
  FDCCHAEBSHHSwSta/1 -> Data Type Conversion/1

== system halout/HAL_OUT/CAN1/FD1_C100_2_0x18FE4A03/FDCCHAEBSRd4BRSta ==
  FDCCHAEBSRd4BRSta : Inport
  Data Type Conversion : DataTypeConversion  OutDataTypeStr=uint8  RndMeth=Round
  CAN1_FDC_CHA_EBSRd4BR_Sta : Outport
  wires:
  Data Type Conversion/1 -> CAN1_FDC_CHA_EBSRd4BR_Sta/1
  FDCCHAEBSRd4BRSta/1 -> Data Type Conversion/1

== system halout/HAL_OUT/CAN1/FD1_C100_3_0xCF103D0/DCDCEnDemand ==
  DCDCEnDemand : Inport
  Data Type Conversion : DataTypeConversion  OutDataTypeStr=uint8  RndMeth=Round
  CAN1_DCDCEnDemand : Outport
  wires:
  Data Type Conversion/1 -> CAN1_DCDCEnDemand/1
  DCDCEnDemand/1 -> Data Type Conversion/1

== system halout/HAL_OUT/CAN1/FD1_C100_3_0xCF103D0/EACSpdDemand ==
  EACSpdDemand : Inport
  Data Type Conversion : DataTypeConversion  OutDataTypeStr=uint16  RndMeth=Round
  convert_out : FVT_lib/hal/convert_out  gain=0.5  offset=-5000
  CAN1_EACSpdDemand : Outport
  wires:
  Data Type Conversion/1 -> CAN1_EACSpdDemand/1
  convert_out/1 -> Data Type Conversion/1
  EACSpdDemand/1 -> convert_out/1

== system halout/HAL_OUT/CAN1/FD1_C100_3_0xCF103D0/EHPSEnDemand ==
  EHPSEnDemand : Inport
  Data Type Conversion : DataTypeConversion  OutDataTypeStr=uint8  RndMeth=Round
  CAN1_EHPSEnDemand : Outport
  wires:
  Data Type Conversion/1 -> CAN1_EHPSEnDemand/1
  EHPSEnDemand/1 -> Data Type Conversion/1

== system halout/HAL_OUT/CAN1/FD1_C100_3_0xCF103D0/EHPSSpdDemand ==
  EHPSSpdDemand : Inport
  Data Type Conversion : DataTypeConversion  OutDataTypeStr=uint16  RndMeth=Round
  convert_out : FVT_lib/hal/convert_out  gain=0.5  offset=-5000
  CAN1_EHPSSpdDemand : Outport
  wires:
  Data Type Conversion/1 -> CAN1_EHPSSpdDemand/1
  convert_out/1 -> Data Type Conversion/1
  EHPSSpdDemand/1 -> convert_out/1

== system halout/HAL_OUT/CAN1/FD1_C100_3_0xCF103D0/FDCCHAEACEnDemandCmd ==
  FDCCHAEACEnDemandCmd : Inport
  Data Type Conversion : DataTypeConversion  OutDataTypeStr=uint8  RndMeth=Round
  CAN1_FDC_CHA_EACEnDemand_Cmd : Outport
  wires:
  Data Type Conversion/1 -> CAN1_FDC_CHA_EACEnDemand_Cmd/1
  FDCCHAEACEnDemandCmd/1 -> Data Type Conversion/1

== system halout/HAL_OUT/CAN1/FD1_CE100_1_0x18FE4EEC/FDCBCMDoorStaSta ==
  FDCBCMDoorStaSta : Inport
  Data Type Conversion : DataTypeConversion  OutDataTypeStr=uint8  RndMeth=Round
  CAN1_FDC_BCM_DoorSta_Sta : Outport
  wires:
  Data Type Conversion/1 -> CAN1_FDC_BCM_DoorSta_Sta/1
  FDCBCMDoorStaSta/1 -> Data Type Conversion/1

== system halout/HAL_OUT/CAN1/GW1_C1000_1_0x18E0FF21/SeatBeltSwitch ==
  SeatBeltSwitch : Inport
  Data Type Conversion : DataTypeConversion  OutDataTypeStr=uint8  RndMeth=Round
  CAN1_SeatBeltSwitch : Outport
  wires:
  Data Type Conversion/1 -> CAN1_SeatBeltSwitch/1
  SeatBeltSwitch/1 -> Data Type Conversion/1

== system halout/HAL_OUT/CAN1/GW1_C100_4_0x18FDA521/OpenStatusOfDoor1 ==
  OpenStatusOfDoor1 : Inport
  Data Type Conversion : DataTypeConversion  OutDataTypeStr=uint8  RndMeth=Round
  CAN1_OpenStatusOfDoor1 : Outport
  wires:
  Data Type Conversion/1 -> CAN1_OpenStatusOfDoor1/1
  OpenStatusOfDoor1/1 -> Data Type Conversion/1

== system halout/HAL_OUT/CAN1/GW1_C100_4_0x18FDA521/OpenStatusOfDoor2 ==
  OpenStatusOfDoor2 : Inport
  Data Type Conversion : DataTypeConversion  OutDataTypeStr=uint8  RndMeth=Round
  CAN1_OpenStatusOfDoor2 : Outport
  wires:
  Data Type Conversion/1 -> CAN1_OpenStatusOfDoor2/1
  OpenStatusOfDoor2/1 -> Data Type Conversion/1

== system halout/HAL_OUT/CAN1/VCU_PDU_Demand_1_0xCF101D0/DCDCRlyEn ==
  DCDCRlyEn : Inport
  Data Type Conversion : DataTypeConversion  OutDataTypeStr=uint8  RndMeth=Round
  CAN1_DCDCRlyEn : Outport
  wires:
  Data Type Conversion/1 -> CAN1_DCDCRlyEn/1
  DCDCRlyEn/1 -> Data Type Conversion/1

== system halout/HAL_OUT/CAN1/VCU_PDU_Demand_1_0xCF101D0/EACRlyEn ==
  EACRlyEn : Inport
  Data Type Conversion : DataTypeConversion  OutDataTypeStr=uint8  RndMeth=Round
  CAN1_EACRlyEn : Outport
  wires:
  Data Type Conversion/1 -> CAN1_EACRlyEn/1
  EACRlyEn/1 -> Data Type Conversion/1

== system halout/HAL_OUT/CAN1/VCU_PDU_Demand_1_0xCF101D0/EHPSRlyEn ==
  EHPSRlyEn : Inport
  Data Type Conversion : DataTypeConversion  OutDataTypeStr=uint8  RndMeth=Round
  CAN1_EHPSRlyEn : Outport
  wires:
  Data Type Conversion/1 -> CAN1_EHPSRlyEn/1
  EHPSRlyEn/1 -> Data Type Conversion/1

== system halout/HAL_OUT/CAN1/VCU_PDU_Demand_1_0xCF101D0/VCULife1 ==
  VCULife1 : Inport
  Data Type Conversion : DataTypeConversion  OutDataTypeStr=uint8  RndMeth=Round
  CAN1_VCULife1 : Outport
  wires:
  Data Type Conversion/1 -> CAN1_VCULife1/1
  VCULife1/1 -> Data Type Conversion/1

== system halout/HAL_OUT/CAN2/FD2_C200_1_0x18F001EF/FDCCHACACPresWarnSta ==
  FDCCHACACPresWarnSta : Inport
  Data Type Conversion : DataTypeConversion  OutDataTypeStr=uint8  RndMeth=Round
  CAN2_FDC_CHA_CACPresWarn_Sta : Outport
  wires:
  Data Type Conversion/1 -> CAN2_FDC_CHA_CACPresWarn_Sta/1
  FDCCHACACPresWarnSta/1 -> Data Type Conversion/1

== system halout/HAL_OUT/CAN2/FD2_C200_1_0x18F001EF/FDCCHACACTempWarnSta ==
  FDCCHACACTempWarnSta : Inport
  Data Type Conversion : DataTypeConversion  OutDataTypeStr=uint8  RndMeth=Round
  CAN2_FDC_CHA_CACTempWarn_Sta : Outport
  wires:
  Data Type Conversion/1 -> CAN2_FDC_CHA_CACTempWarn_Sta/1
  FDCCHACACTempWarnSta/1 -> Data Type Conversion/1

== system halout/HAL_OUT/CAN2/FD2_C20_0_0x210/APSExitCondition ==
  APSExitCondition : Inport
  Data Type Conversion : DataTypeConversion  OutDataTypeStr=uint8  RndMeth=Round
  CAN2_APS_ExitCondition : Outport
  wires:
  Data Type Conversion/1 -> CAN2_APS_ExitCondition/1
  APSExitCondition/1 -> Data Type Conversion/1

== system halout/HAL_OUT/CAN2/FD2_C20_0_0x210/APSRQDisplay ==
  APSRQDisplay : Inport
  Data Type Conversion : DataTypeConversion  OutDataTypeStr=uint8  RndMeth=Round
  CAN2_APS_RQ_Display : Outport
  wires:
  Data Type Conversion/1 -> CAN2_APS_RQ_Display/1
  APSRQDisplay/1 -> Data Type Conversion/1

== system halout/HAL_OUT/CAN2/FD2_C20_0_0x210/APSSWVer ==
  APSSWVer : Inport
  Data Type Conversion : DataTypeConversion  OutDataTypeStr=uint8  RndMeth=Round
  CAN2_APS_SW_Ver : Outport
  wires:
  Data Type Conversion/1 -> CAN2_APS_SW_Ver/1
  APSSWVer/1 -> Data Type Conversion/1

== system halout/HAL_OUT/CAN2/FD2_C20_0_0x210/APSStaSystem ==
  APSStaSystem : Inport
  Data Type Conversion : DataTypeConversion  OutDataTypeStr=uint8  RndMeth=Round
  CAN2_APS_Sta_System : Outport
  wires:
  Data Type Conversion/1 -> CAN2_APS_Sta_System/1
  APSStaSystem/1 -> Data Type Conversion/1

== system halout/HAL_OUT/CAN2/FD2_C20_0_0x210/CAASSta ==
  CAASSta : Inport
  Data Type Conversion : DataTypeConversion  OutDataTypeStr=uint8  RndMeth=Round
  CAN2_CAAS_Sta : Outport
  wires:
  Data Type Conversion/1 -> CAN2_CAAS_Sta/1
  CAASSta/1 -> Data Type Conversion/1

== system halout/HAL_OUT/CAN2/FD2_C20_0_0x210/FDCVCURegenLimIndSta ==
  FDCVCURegenLimIndSta : Inport
  Data Type Conversion : DataTypeConversion  OutDataTypeStr=uint8  RndMeth=Round
  CAN2_FDC_VCU_RegenLimInd_Sta : Outport
  wires:
  Data Type Conversion/1 -> CAN2_FDC_VCU_RegenLimInd_Sta/1
  FDCVCURegenLimIndSta/1 -> Data Type Conversion/1

== system halout/HAL_OUT/CAN2/FD2_C20_0_0x210/FDCVCURegenModeSta ==
  FDCVCURegenModeSta : Inport
  Data Type Conversion : DataTypeConversion  OutDataTypeStr=uint8  RndMeth=Round
  CAN2_FDC_VCU_RegenMode_Sta : Outport
  wires:
  Data Type Conversion/1 -> CAN2_FDC_VCU_RegenMode_Sta/1
  FDCVCURegenModeSta/1 -> Data Type Conversion/1

== system halout/HAL_OUT/CAN2/FD2_C20_0_0x210/FDCVCUSmartEcoSpdLimSta ==
  FDCVCUSmartEcoSpdLimSta : Inport
  Data Type Conversion : DataTypeConversion  OutDataTypeStr=uint8  RndMeth=Round
  CAN2_FDC_VCU_SmartEcoSpdLim_Sta : Outport
  wires:
  Data Type Conversion/1 -> CAN2_FDC_VCU_SmartEcoSpdLim_Sta/1
  FDCVCUSmartEcoSpdLimSta/1 -> Data Type Conversion/1

== system halout/HAL_OUT/CAN2/FD2_C20_0_0x210/FDCVCUSmartEcoSta ==
  FDCVCUSmartEcoSta : Inport
  Data Type Conversion : DataTypeConversion  OutDataTypeStr=uint8  RndMeth=Round
  CAN2_FDC_VCU_SmartEco_Sta : Outport
  wires:
  Data Type Conversion/1 -> CAN2_FDC_VCU_SmartEco_Sta/1
  FDCVCUSmartEcoSta/1 -> Data Type Conversion/1

== system halout/HAL_OUT/CAN2/FD2_C20_0_0x210/FDCVMCSetSpdDispSta ==
  FDCVMCSetSpdDispSta : Inport
  Data Type Conversion : DataTypeConversion  OutDataTypeStr=uint8  RndMeth=Round
  CAN2_FDC_VMC_SetSpdDisp_Sta : Outport
  wires:
  Data Type Conversion/1 -> CAN2_FDC_VMC_SetSpdDisp_Sta/1
  FDCVMCSetSpdDispSta/1 -> Data Type Conversion/1

== system halout/HAL_OUT/CAN2/FD2_C20_0_0x210/FDCVMCSetSpdSta ==
  FDCVMCSetSpdSta : Inport
  Data Type Conversion : DataTypeConversion  OutDataTypeStr=uint8  RndMeth=Round
  CAN2_FDC_VMC_SetSpd_Sta : Outport
  wires:
  Data Type Conversion/1 -> CAN2_FDC_VMC_SetSpd_Sta/1
  FDCVMCSetSpdSta/1 -> Data Type Conversion/1

== system halout/HAL_OUT/CAN2/FD2_C20_0_0x210/FDCVMCSpdCtrlModeSta ==
  FDCVMCSpdCtrlModeSta : Inport
  Data Type Conversion : DataTypeConversion  OutDataTypeStr=uint8  RndMeth=Round
  CAN2_FDC_VMC_SpdCtrlMode_Sta : Outport
  wires:
  Data Type Conversion/1 -> CAN2_FDC_VMC_SpdCtrlMode_Sta/1
  FDCVMCSpdCtrlModeSta/1 -> Data Type Conversion/1

== system halout/HAL_OUT/CAN2/FD2_C20_0_0x210/FDCVMCSpdCtrlSta ==
  FDCVMCSpdCtrlSta : Inport
  Data Type Conversion : DataTypeConversion  OutDataTypeStr=uint8  RndMeth=Round
  CAN2_FDC_VMC_SpdCtrl_Sta : Outport
  wires:
  Data Type Conversion/1 -> CAN2_FDC_VMC_SpdCtrl_Sta/1
  FDCVMCSpdCtrlSta/1 -> Data Type Conversion/1

== system halout/HAL_OUT/CAN2/FD2_C20_0_0x210/PASAFCL ==
  PASAFCL : Inport
  Data Type Conversion : DataTypeConversion  OutDataTypeStr=uint8  RndMeth=Round
  CAN2_PAS_A_FCL : Outport
  wires:
  Data Type Conversion/1 -> CAN2_PAS_A_FCL/1
  PASAFCL/1 -> Data Type Conversion/1

== system halout/HAL_OUT/CAN2/FD2_C20_0_0x210/PASAFCR ==
  PASAFCR : Inport
  Data Type Conversion : DataTypeConversion  OutDataTypeStr=uint8  RndMeth=Round
  CAN2_PAS_A_FCR : Outport
  wires:
  Data Type Conversion/1 -> CAN2_PAS_A_FCR/1
  PASAFCR/1 -> Data Type Conversion/1

== system halout/HAL_OUT/CAN2/FD2_C20_0_0x210/PASAFML ==
  PASAFML : Inport
  Data Type Conversion : DataTypeConversion  OutDataTypeStr=uint8  RndMeth=Round
  CAN2_PAS_A_FML : Outport
  wires:
  Data Type Conversion/1 -> CAN2_PAS_A_FML/1
  PASAFML/1 -> Data Type Conversion/1

== system halout/HAL_OUT/CAN2/FD2_C20_0_0x210/PASAFMR ==
  PASAFMR : Inport
  Data Type Conversion : DataTypeConversion  OutDataTypeStr=uint8  RndMeth=Round
  CAN2_PAS_A_FMR : Outport
  wires:
  Data Type Conversion/1 -> CAN2_PAS_A_FMR/1
  PASAFMR/1 -> Data Type Conversion/1

== system halout/HAL_OUT/CAN2/FD2_C20_0_0x210/PASARCL ==
  PASARCL : Inport
  Data Type Conversion : DataTypeConversion  OutDataTypeStr=uint8  RndMeth=Round
  CAN2_PAS_A_RCL : Outport
  wires:
  Data Type Conversion/1 -> CAN2_PAS_A_RCL/1
  PASARCL/1 -> Data Type Conversion/1

== system halout/HAL_OUT/CAN2/FD2_C20_0_0x210/PASARCR ==
  PASARCR : Inport
  Data Type Conversion : DataTypeConversion  OutDataTypeStr=uint8  RndMeth=Round
  CAN2_PAS_A_RCR : Outport
  wires:
  Data Type Conversion/1 -> CAN2_PAS_A_RCR/1
  PASARCR/1 -> Data Type Conversion/1

== system halout/HAL_OUT/CAN2/FD2_C20_0_0x210/PASARML ==
  PASARML : Inport
  Data Type Conversion : DataTypeConversion  OutDataTypeStr=uint8  RndMeth=Round
  CAN2_PAS_A_RML : Outport
  wires:
  Data Type Conversion/1 -> CAN2_PAS_A_RML/1
  PASARML/1 -> Data Type Conversion/1

== system halout/HAL_OUT/CAN2/FD2_C20_0_0x210/PASARMR ==
  PASARMR : Inport
  Data Type Conversion : DataTypeConversion  OutDataTypeStr=uint8  RndMeth=Round
  CAN2_PAS_A_RMR : Outport
  wires:
  Data Type Conversion/1 -> CAN2_PAS_A_RMR/1
  PASARMR/1 -> Data Type Conversion/1

== system halout/HAL_OUT/CAN2/FD2_C20_0_0x210/PASChime ==
  PASChime : Inport
  Data Type Conversion : DataTypeConversion  OutDataTypeStr=uint8  RndMeth=Round
  CAN2_PAS_Chime : Outport
  wires:
  Data Type Conversion/1 -> CAN2_PAS_Chime/1
  PASChime/1 -> Data Type Conversion/1

== system halout/HAL_OUT/CAN2/FD2_C20_0_0x210/PASDFCL ==
  PASDFCL : Inport
  Data Type Conversion : DataTypeConversion  OutDataTypeStr=uint8  RndMeth=Round
  CAN2_PAS_D_FCL : Outport
  wires:
  Data Type Conversion/1 -> CAN2_PAS_D_FCL/1
  PASDFCL/1 -> Data Type Conversion/1

== system halout/HAL_OUT/CAN2/FD2_C20_0_0x210/PASDFCR ==
  PASDFCR : Inport
  Data Type Conversion : DataTypeConversion  OutDataTypeStr=uint8  RndMeth=Round
  CAN2_PAS_D_FCR : Outport
  wires:
  Data Type Conversion/1 -> CAN2_PAS_D_FCR/1
  PASDFCR/1 -> Data Type Conversion/1

== system halout/HAL_OUT/CAN2/FD2_C20_0_0x210/PASDFML ==
  PASDFML : Inport
  Data Type Conversion : DataTypeConversion  OutDataTypeStr=uint8  RndMeth=Round
  CAN2_PAS_D_FML : Outport
  wires:
  Data Type Conversion/1 -> CAN2_PAS_D_FML/1
  PASDFML/1 -> Data Type Conversion/1

== system halout/HAL_OUT/CAN2/FD2_C20_0_0x210/PASDFMR ==
  PASDFMR : Inport
  Data Type Conversion : DataTypeConversion  OutDataTypeStr=uint8  RndMeth=Round
  CAN2_PAS_D_FMR : Outport
  wires:
  Data Type Conversion/1 -> CAN2_PAS_D_FMR/1
  PASDFMR/1 -> Data Type Conversion/1

== system halout/HAL_OUT/CAN2/FD2_C20_0_0x210/PASDRCL ==
  PASDRCL : Inport
  Data Type Conversion : DataTypeConversion  OutDataTypeStr=uint8  RndMeth=Round
  CAN2_PAS_D_RCL : Outport
  wires:
  Data Type Conversion/1 -> CAN2_PAS_D_RCL/1
  PASDRCL/1 -> Data Type Conversion/1

== system halout/HAL_OUT/CAN2/FD2_C20_0_0x210/PASDRCR ==
  PASDRCR : Inport
  Data Type Conversion : DataTypeConversion  OutDataTypeStr=uint8  RndMeth=Round
  CAN2_PAS_D_RCR : Outport
  wires:
  Data Type Conversion/1 -> CAN2_PAS_D_RCR/1
  PASDRCR/1 -> Data Type Conversion/1

== system halout/HAL_OUT/CAN2/FD2_C20_0_0x210/PASDRML ==
  PASDRML : Inport
  Data Type Conversion : DataTypeConversion  OutDataTypeStr=uint8  RndMeth=Round
  CAN2_PAS_D_RML : Outport
  wires:
  Data Type Conversion/1 -> CAN2_PAS_D_RML/1
  PASDRML/1 -> Data Type Conversion/1

== system halout/HAL_OUT/CAN2/FD2_C20_0_0x210/PASDRMR ==
  PASDRMR : Inport
  Data Type Conversion : DataTypeConversion  OutDataTypeStr=uint8  RndMeth=Round
  CAN2_PAS_D_RMR : Outport
  wires:
  Data Type Conversion/1 -> CAN2_PAS_D_RMR/1
  PASDRMR/1 -> Data Type Conversion/1

== system halout/HAL_OUT/CAN2/FD2_C20_0_0x210/PASSNSRLayout ==
  PASSNSRLayout : Inport
  Data Type Conversion : DataTypeConversion  OutDataTypeStr=uint8  RndMeth=Round
  CAN2_PAS_SNSR_Layout : Outport
  wires:
  Data Type Conversion/1 -> CAN2_PAS_SNSR_Layout/1
  PASSNSRLayout/1 -> Data Type Conversion/1

== system halout/HAL_OUT/CAN2/FD2_C20_0_0x210/USSStaFCL ==
  USSStaFCL : Inport
  Data Type Conversion : DataTypeConversion  OutDataTypeStr=uint8  RndMeth=Round
  CAN2_USS_Sta_FCL : Outport
  wires:
  Data Type Conversion/1 -> CAN2_USS_Sta_FCL/1
  USSStaFCL/1 -> Data Type Conversion/1

== system halout/HAL_OUT/CAN2/FD2_C20_0_0x210/USSStaFCR ==
  USSStaFCR : Inport
  Data Type Conversion : DataTypeConversion  OutDataTypeStr=uint8  RndMeth=Round
  CAN2_USS_Sta_FCR : Outport
  wires:
  Data Type Conversion/1 -> CAN2_USS_Sta_FCR/1
  USSStaFCR/1 -> Data Type Conversion/1

== system halout/HAL_OUT/CAN2/FD2_C20_0_0x210/USSStaFLL ==
  USSStaFLL : Inport
  Data Type Conversion : DataTypeConversion  OutDataTypeStr=uint8  RndMeth=Round
  CAN2_USS_Sta_FLL : Outport
  wires:
  Data Type Conversion/1 -> CAN2_USS_Sta_FLL/1
  USSStaFLL/1 -> Data Type Conversion/1

== system halout/HAL_OUT/CAN2/FD2_C20_0_0x210/USSStaFLR ==
  USSStaFLR : Inport
  Data Type Conversion : DataTypeConversion  OutDataTypeStr=uint8  RndMeth=Round
  CAN2_USS_Sta_FLR : Outport
  wires:
  Data Type Conversion/1 -> CAN2_USS_Sta_FLR/1
  USSStaFLR/1 -> Data Type Conversion/1

== system halout/HAL_OUT/CAN2/FD2_C20_0_0x210/USSStaFML ==
  USSStaFML : Inport
  Data Type Conversion : DataTypeConversion  OutDataTypeStr=uint8  RndMeth=Round
  CAN2_USS_Sta_FML : Outport
  wires:
  Data Type Conversion/1 -> CAN2_USS_Sta_FML/1
  USSStaFML/1 -> Data Type Conversion/1

== system halout/HAL_OUT/CAN2/FD2_C20_0_0x210/USSStaFMR ==
  USSStaFMR : Inport
  Data Type Conversion : DataTypeConversion  OutDataTypeStr=uint8  RndMeth=Round
  CAN2_USS_Sta_FMR : Outport
  wires:
  Data Type Conversion/1 -> CAN2_USS_Sta_FMR/1
  USSStaFMR/1 -> Data Type Conversion/1

== system halout/HAL_OUT/CAN2/FD2_C20_0_0x210/USSStaRCL ==
  USSStaRCL : Inport
  Data Type Conversion : DataTypeConversion  OutDataTypeStr=uint8  RndMeth=Round
  CAN2_USS_Sta_RCL : Outport
  wires:
  Data Type Conversion/1 -> CAN2_USS_Sta_RCL/1
  USSStaRCL/1 -> Data Type Conversion/1

== system halout/HAL_OUT/CAN2/FD2_C20_0_0x210/USSStaRCR ==
  USSStaRCR : Inport
  Data Type Conversion : DataTypeConversion  OutDataTypeStr=uint8  RndMeth=Round
  CAN2_USS_Sta_RCR : Outport
  wires:
  Data Type Conversion/1 -> CAN2_USS_Sta_RCR/1
  USSStaRCR/1 -> Data Type Conversion/1

== system halout/HAL_OUT/CAN2/FD2_C20_0_0x210/USSStaRLL ==
  USSStaRLL : Inport
  Data Type Conversion : DataTypeConversion  OutDataTypeStr=uint8  RndMeth=Round
  CAN2_USS_Sta_RLL : Outport
  wires:
  Data Type Conversion/1 -> CAN2_USS_Sta_RLL/1
  USSStaRLL/1 -> Data Type Conversion/1

== system halout/HAL_OUT/CAN2/FD2_C20_0_0x210/USSStaRLR ==
  USSStaRLR : Inport
  Data Type Conversion : DataTypeConversion  OutDataTypeStr=uint8  RndMeth=Round
  CAN2_USS_Sta_RLR : Outport
  wires:
  Data Type Conversion/1 -> CAN2_USS_Sta_RLR/1
  USSStaRLR/1 -> Data Type Conversion/1

== system halout/HAL_OUT/CAN2/FD2_C20_0_0x210/USSStaRML ==
  USSStaRML : Inport
  Data Type Conversion : DataTypeConversion  OutDataTypeStr=uint8  RndMeth=Round
  CAN2_USS_Sta_RML : Outport
  wires:
  Data Type Conversion/1 -> CAN2_USS_Sta_RML/1
  USSStaRML/1 -> Data Type Conversion/1
